simulink model "cUniforme"  (R2015a)
settings: Solver=VariableStepDiscrete  StartTime=0.0  StopTime=10.0  RelTol=1e-3
settings Model: Creator=Javi  LastModifiedBy=Javi

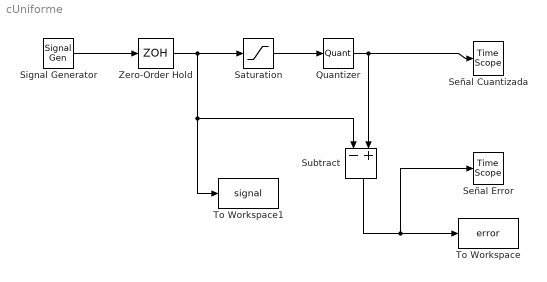
== system cUniforme ==
  Quantizer : Quantizer  QuantizationInterval=2/16  LinearizeAsGain=off
  Saturation : Saturate  UpperLimit=1  LowerLimit=-1
  Señal Cuantizada : TimeScope
  Señal Error : TimeScope
  Signal Generator : SignalGenerator  Units=rad/sec
  Subtract : Sum  Inputs=-+
  To Workspace : ToWorkspace  VariableName=error  SampleTime=-1
      settings: Save2DSignal=2-D array (concatenate along first dimension)
  To Workspace1 : ToWorkspace  VariableName=signal  SampleTime=-1
      settings: Save2DSignal=2-D array (concatenate along first dimension)
  Zero-Order Hold : ZeroOrderHold  SampleTime=0.01
  wires:
  Zero-Order Hold/1 -> Subtract/1, To Workspace1/1, Saturation/1
  Saturation/1 -> Quantizer/1
  Quantizer/1 -> Subtract/2, Señal Cuantizada/1
  Subtract/1 -> Señal Error/1, To Workspace/1
  Signal Generator/1 -> Zero-Order Hold/1
